simulink model "ssc_auto_ev_20b"  (R2020b)
settings: Solver=VariableStepAuto  StartTime=0.0  StopTime=200  RelTol=1e-3  AbsTol=1e-3
PreLoadFcn:
  | % Simulation parameters
  | dt = 0.01;
  | 
  | % Battery cell parameters
  | ssc_lithium_cell_1RC_ini
  | Nseries = 100;
  | Nparallel = 10;
  | 
  | % Motor parameters
  | max_torque = 220;
  | max_power = 80e3;
  | 
  | % Vehicle parameters
  | vehicle_mass = 4000;
  | wheel_radius = 0.35;
  | area = 5;
  | drag_coefficient = 0.25;
  | air_density = 1.225;
  | gravity = 9.81;
  | rolling_res_ratio = 0.015;
  | 
  | % Differential drive parameters
  | gear_ratio = 12;
  | 
  | % Simplified braking system parameters
  | force_max_pedal = 500;
  | braking_torque_to_pedal_force_ratio = -16;
  | 
  | % Vehicle controller parameters
  | hill_hold_max_speed = 0.5;
  | 
  | % Water properties for cooling circuit
  | load WaterProperties
  | 
  | % Input signals for Signal Editor block
  | load ssc_auto_ev_Inputs
values from neighbouring files (symbols this model uses):
  C1_LUT = [1913.6 4625.7 23306 10736 18036 12251 9022.9 12447 18872 40764 18721 33630 ... (21 elements, 7x3)]    [ssc_auto_ev_param.mat]
  Capacity_LUT = [28.0081 27.625 27.6392]    [ssc_auto_ev_param.mat]
  cell_Cp_heat = 810.5328    [ssc_auto_ev_param.mat]
  cell_mass = 1    [ssc_auto_ev_param.mat]
  Em_LUT = [3.4966 3.5519 3.6183 3.7066 3.9131 4.0748 4.1923 3.5057 3.566 3.6337 3.7127 3.9259 ... (21 elements, 7x3)]    [ssc_auto_ev_param.mat]
  Qe_init = 15.6845    [ssc_auto_ev_param.mat]
  R0_LUT = [0.0117 0.011 0.0114 0.0107 0.0107 0.0113 0.0116 0.0085 0.0085 0.0087 0.0082 0.0083 ... (21 elements, 7x3)]    [ssc_auto_ev_param.mat]
  R1_LUT = [0.0109 0.0069 0.0047 0.0034 0.0033 0.0033 0.0028 0.0029 0.0024 0.0026 0.0016 0.0023 ... (21 elements, 7x3)]    [ssc_auto_ev_param.mat]
  SOC_LUT = [0 0.1 0.25 0.5 0.75 0.9 1]    [ssc_auto_ev_param.mat]
  T_init = 293.15    [ssc_auto_ev_param.mat]
  Temperature_LUT = [278.15 293.15 313.15]    [ssc_auto_ev_param.mat]
undefined symbols (not defined in the file or in its folder): DiscIntNeverNeededParam, K, Lambda, tau, x0
libraries: fl_lib x656, nesl_utility x86, simulink x21, LiBatteryElements_lib x16, SignalEditorBlockLib x4, simulink_extras x4
(part 11 of 13)

== system ssc_auto_ev_20b/Step 3: Ungroup and Redraw/Port 1 Interface1/Interface/Continuous ==
  through2 : Inport
  through1 : Inport  Port=2
  1/thermalMass : Gain  Gain=1/thermalMass  SaturateOnIntegerOverflow=on  OutDataTypeStr=Inherit: Same as input  ParamDataTypeStr=Inherit: Same as input
  Integrator : Integrator  InitialCondition=T0
  Prediction : Subsystem  Commented=through  mask(Prediction (discrete->continuous)){h2=h2}
      mask prompts: h2 "physmod:simscape:couplers:SimscapeNetworkCouplersLib:PortUDiscreteSampleTimes_MP"
      mask help: physmod:simscape:couplers:SimscapeNetworkCouplersLib:Predictiondiscretecontinuous_MD
  Smoothing : Subsystem  Commented=through  mask(Smoothing (continuous->discrete)){tsSmoothing=tsSmoothing, smoothing0=T0}
      mask prompts: tsSmoothing "physmod:simscape:couplers:SimscapeNetworkCouplersLib:SmoothingTimeConstants_MP"; smoothing0 "physmod:simscape:couplers:SimscapeNetworkCouplersLib:InitialOutput_MP"
      mask help: physmod:simscape:couplers:SimscapeNetworkCouplersLib:Smoothingcontinuousdiscrete_MD
  Sum : Sum  InputSameDT=on  SaturateOnIntegerOverflow=on  OutDataTypeStr=Inherit: Same as first input
  across2 : Outport
  across1 : Outport  Port=2
  wires:
  Integrator/1 -> Smoothing/1(u), across1/1
  1/thermalMass/1 -> Integrator/1
  Sum/1 -> 1/thermalMass/1
  Smoothing/1(y) -> across2/1
  Prediction/1(y) -> Sum/2
  through1/1 -> Sum/1
  through2/1 -> Prediction/1(u)

== system ssc_auto_ev_20b/Step 3: Ungroup and Redraw/Port 1 Interface1/Interface/Discrete ==
  through2 : Inport
  through1 : Inport  Port=2
  1/thermalMass : Gain  Gain=1/thermalMass  SaturateOnIntegerOverflow=on  OutDataTypeStr=Inherit: Same as input  ParamDataTypeStr=Inherit: Same as input
  Integrator : DiscreteIntegrator  InitialCondition=T0  SampleTime=h1  ICPrevOutput=DiscIntNeverNeededParam  ICPrevScaledInput=DiscIntNeverNeededParam
  Prediction : Subsystem  Commented=through  mask(Prediction (slow->fast)){h2=h2, h1=h1}
      mask prompts: h2 "physmod:simscape:couplers:SimscapeNetworkCouplersLib:PortUDiscreteSampleTimes_MP"; h1 "physmod:simscape:couplers:SimscapeNetworkCouplersLib:PortYDiscreteSampleTimes_MP"
      mask help: physmod:simscape:couplers:SimscapeNetworkCouplersLib:Predictionslowfast_MD
  Smoothing : Subsystem  Commented=through  mask(Smoothing (fast->slow)){nSmooth=nSmooth, h1=h1, smoothing0=T0}
      mask prompts: nSmooth "physmod:simscape:couplers:SimscapeNetworkCouplersLib:NumberOfSamplesOverWhichToSmooth_MP"; h1 "physmod:simscape:couplers:SimscapeNetworkCouplersLib:PortUDiscreteSampleTimes_MP"; smoothing0 "physmod:simscape:couplers:SimscapeNetworkCouplersLib:InitialOutput_MP"
      mask help: physmod:simscape:couplers:SimscapeNetworkCouplersLib:Smoothingfastslow_MD
  Sum : Sum  InputSameDT=on  SaturateOnIntegerOverflow=on  OutDataTypeStr=Inherit: Same as first input
  across2 : Outport
  across1 : Outport  Port=2
  wires:
  1/thermalMass/1 -> Integrator/1
  Sum/1 -> 1/thermalMass/1
  Integrator/1 -> Smoothing/1(u), across1/1
  Smoothing/1(y) -> across2/1
  Prediction/1(y) -> Sum/2
  through2/1 -> Prediction/1(u)
  through1/1 -> Sum/1

== system ssc_auto_ev_20b/Step 3: Ungroup and Redraw/Port 1 Interface2/Interface/Continuous ==
  through2 : Inport
  through1 : Inport  Port=2
  1/thermalMass : Gain  Gain=1/thermalMass  SaturateOnIntegerOverflow=on  OutDataTypeStr=Inherit: Same as input  ParamDataTypeStr=Inherit: Same as input
  Integrator : Integrator  InitialCondition=T0
  Prediction : Subsystem  Commented=through  mask(Prediction (discrete->continuous)){h2=h2}
      mask prompts: h2 "physmod:simscape:couplers:SimscapeNetworkCouplersLib:PortUDiscreteSampleTimes_MP"
      mask help: physmod:simscape:couplers:SimscapeNetworkCouplersLib:Predictiondiscretecontinuous_MD
  Smoothing : Subsystem  Commented=through  mask(Smoothing (continuous->discrete)){tsSmoothing=tsSmoothing, smoothing0=T0}
      mask prompts: tsSmoothing "physmod:simscape:couplers:SimscapeNetworkCouplersLib:SmoothingTimeConstants_MP"; smoothing0 "physmod:simscape:couplers:SimscapeNetworkCouplersLib:InitialOutput_MP"
      mask help: physmod:simscape:couplers:SimscapeNetworkCouplersLib:Smoothingcontinuousdiscrete_MD
  Sum : Sum  InputSameDT=on  SaturateOnIntegerOverflow=on  OutDataTypeStr=Inherit: Same as first input
  across2 : Outport
  across1 : Outport  Port=2
  wires:
  through2/1 -> Prediction/1(u)
  through1/1 -> Sum/1
  Prediction/1(y) -> Sum/2
  Smoothing/1(y) -> across2/1
  Sum/1 -> 1/thermalMass/1
  1/thermalMass/1 -> Integrator/1
  Integrator/1 -> across1/1, Smoothing/1(u)

== system ssc_auto_ev_20b/Step 3: Ungroup and Redraw/Port 1 Interface2/Interface/Discrete ==
  through2 : Inport
  through1 : Inport  Port=2
  1/thermalMass : Gain  Gain=1/thermalMass  SaturateOnIntegerOverflow=on  OutDataTypeStr=Inherit: Same as input  ParamDataTypeStr=Inherit: Same as input
  Integrator : DiscreteIntegrator  InitialCondition=T0  SampleTime=h1  ICPrevOutput=DiscIntNeverNeededParam  ICPrevScaledInput=DiscIntNeverNeededParam
  Prediction : Subsystem  Commented=through  mask(Prediction (slow->fast)){h2=h2, h1=h1}
      mask prompts: h2 "physmod:simscape:couplers:SimscapeNetworkCouplersLib:PortUDiscreteSampleTimes_MP"; h1 "physmod:simscape:couplers:SimscapeNetworkCouplersLib:PortYDiscreteSampleTimes_MP"
      mask help: physmod:simscape:couplers:SimscapeNetworkCouplersLib:Predictionslowfast_MD
  Smoothing : Subsystem  Commented=through  mask(Smoothing (fast->slow)){nSmooth=nSmooth, h1=h1, smoothing0=T0}
      mask prompts: nSmooth "physmod:simscape:couplers:SimscapeNetworkCouplersLib:NumberOfSamplesOverWhichToSmooth_MP"; h1 "physmod:simscape:couplers:SimscapeNetworkCouplersLib:PortUDiscreteSampleTimes_MP"; smoothing0 "physmod:simscape:couplers:SimscapeNetworkCouplersLib:InitialOutput_MP"
      mask help: physmod:simscape:couplers:SimscapeNetworkCouplersLib:Smoothingfastslow_MD
  Sum : Sum  InputSameDT=on  SaturateOnIntegerOverflow=on  OutDataTypeStr=Inherit: Same as first input
  across2 : Outport
  across1 : Outport  Port=2
  wires:
  through1/1 -> Sum/1
  through2/1 -> Prediction/1(u)
  Prediction/1(y) -> Sum/2
  Smoothing/1(y) -> across2/1
  Integrator/1 -> across1/1, Smoothing/1(u)
  Sum/1 -> 1/thermalMass/1
  1/thermalMass/1 -> Integrator/1

== system ssc_auto_ev_20b/Step 3: Ungroup and Redraw/Port 1 Interface3/Interface/Continuous ==
  across2 : Inport
  through1 : Inport  Port=2
  -1 : Gain  Gain=-1  SaturateOnIntegerOverflow=on  OutDataTypeStr=Inherit: Same as input  ParamDataTypeStr=Inherit: Same as input
  1/tau : Gain  Gain=1/tau  SaturateOnIntegerOverflow=on  OutDataTypeStr=Inherit: Same as input  ParamDataTypeStr=Inherit: Same as input
  1/tau1 : Gain  Gain=1/tau  SaturateOnIntegerOverflow=on  OutDataTypeStr=Inherit: Same as input  ParamDataTypeStr=Inherit: Same as input
  Integrator : Integrator  InitialCondition=i0
  Integrator1 : Integrator  InitialCondition=v0
  Prediction : Subsystem  Commented=through  mask(Prediction (discrete->continuous)){h2=h2}
      mask prompts: h2 "physmod:simscape:couplers:SimscapeNetworkCouplersLib:PortUDiscreteSampleTimes_MP"
      mask help: physmod:simscape:couplers:SimscapeNetworkCouplersLib:Predictiondiscretecontinuous_MD
  Smoothing : Subsystem  Commented=through  mask(Smoothing (continuous->discrete)){tsSmoothing=tsSmoothing, smoothing0=i0}
      mask prompts: tsSmoothing "physmod:simscape:couplers:SimscapeNetworkCouplersLib:SmoothingTimeConstants_MP"; smoothing0 "physmod:simscape:couplers:SimscapeNetworkCouplersLib:InitialOutput_MP"
      mask help: physmod:simscape:couplers:SimscapeNetworkCouplersLib:Smoothingcontinuousdiscrete_MD
  Sum : Sum  Inputs=|+-  InputSameDT=on  SaturateOnIntegerOverflow=on  OutDataTypeStr=Inherit: Same as first input
  Sum1 : Sum  Inputs=|+-  InputSameDT=on  SaturateOnIntegerOverflow=on  OutDataTypeStr=Inherit: Same as first input
  through2 : Outport
  across1 : Outport  Port=2
  wires:
  across2/1 -> Prediction/1(u)
  Smoothing/1(y) -> -1/1
  1/tau/1 -> Integrator/1
  Sum/1 -> 1/tau/1
  Integrator/1 -> Smoothing/1(u), Sum/2
  through1/1 -> Sum/1
  Integrator1/1 -> Sum1/2, across1/1
  1/tau1/1 -> Integrator1/1
  Sum1/1 -> 1/tau1/1
  Prediction/1(y) -> Sum1/1
  -1/1 -> through2/1

== system ssc_auto_ev_20b/Step 3: Ungroup and Redraw/Port 1 Interface3/Interface/Discrete ==
  across2 : Inport
  through1 : Inport  Port=2
  -1 : Gain  Gain=-1  SaturateOnIntegerOverflow=on  OutDataTypeStr=Inherit: Same as input  ParamDataTypeStr=Inherit: Same as input
  1/tau : Gain  Gain=1/tau  SaturateOnIntegerOverflow=on  OutDataTypeStr=Inherit: Same as input  ParamDataTypeStr=Inherit: Same as input
  1/tau1 : Gain  Gain=1/tau  SaturateOnIntegerOverflow=on  OutDataTypeStr=Inherit: Same as input  ParamDataTypeStr=Inherit: Same as input
  Integrator/1 : DiscreteIntegrator  InitialCondition=v0  SampleTime=h1  ICPrevOutput=DiscIntNeverNeededParam  ICPrevScaledInput=DiscIntNeverNeededParam
  Integrator/2 : DiscreteIntegrator  InitialCondition=i0  SampleTime=h1  ICPrevOutput=DiscIntNeverNeededParam  ICPrevScaledInput=DiscIntNeverNeededParam
  Prediction : Subsystem  Commented=through  mask(Prediction (slow->fast)){h2=h2, h1=h1}
      mask prompts: h2 "physmod:simscape:couplers:SimscapeNetworkCouplersLib:PortUDiscreteSampleTimes_MP"; h1 "physmod:simscape:couplers:SimscapeNetworkCouplersLib:PortYDiscreteSampleTimes_MP"
      mask help: physmod:simscape:couplers:SimscapeNetworkCouplersLib:Predictionslowfast_MD
  Smoothing : Subsystem  Commented=through  mask(Smoothing (fast->slow)){nSmooth=nSmooth, h1=h1, smoothing0=i0}
      mask prompts: nSmooth "physmod:simscape:couplers:SimscapeNetworkCouplersLib:NumberOfSamplesOverWhichToSmooth_MP"; h1 "physmod:simscape:couplers:SimscapeNetworkCouplersLib:PortUDiscreteSampleTimes_MP"; smoothing0 "physmod:simscape:couplers:SimscapeNetworkCouplersLib:InitialOutput_MP"
      mask help: physmod:simscape:couplers:SimscapeNetworkCouplersLib:Smoothingfastslow_MD
  Sum : Sum  Inputs=|+-  InputSameDT=on  SaturateOnIntegerOverflow=on  OutDataTypeStr=Inherit: Same as first input
  Sum1 : Sum  Inputs=|+-  InputSameDT=on  SaturateOnIntegerOverflow=on  OutDataTypeStr=Inherit: Same as first input
  through2 : Outport
  across1 : Outport  Port=2
  wires:
  across2/1 -> Prediction/1(u)
  Smoothing/1(y) -> -1/1
  Prediction/1(y) -> Sum1/1
  Sum1/1 -> 1/tau1/1
  Integrator/1/1 -> across1/1, Sum1/2
  Integrator/2/1 -> Smoothing/1(u), Sum/2
  Sum/1 -> 1/tau/1
  1/tau1/1 -> Integrator/1/1
  1/tau/1 -> Integrator/2/1
  through1/1 -> Sum/1
  -1/1 -> through2/1

== system ssc_auto_ev_20b/Step 3: Ungroup and Redraw/Vehicle Dynamics/Brake Torque/Smooth Sign ==
  1 : fl_lib/Physical Signals/Sources/PS Constant  constant=1
      settings: SourceProductBaseCode=PW,SS,VE
  2 : fl_lib/Physical Signals/Functions/PS Gain  gain=2 1/(rad/s)
      settings: SourceProductBaseCode=PW,SS,VE
  PS Add : fl_lib/Physical Signals/Functions/PS Add
      settings: SourceProductBaseCode=PW,SS,VE
  PS Subtract : fl_lib/Physical Signals/Functions/PS Subtract
      settings: SourceProductBaseCode=PW,SS,VE
  exp(2x) : fl_lib/Physical Signals/Functions/PS Math Function  fcn_choice=foundation.enum.math_function.exp
      settings: SourceProductBaseCode=PW,SS,VE
  tanh(x) : fl_lib/Physical Signals/Functions/PS Divide
      settings: SourceProductBaseCode=PW,SS,VE
  x : PMIOPort  Side=Left
  y : PMIOPort  Port=2  Side=Right
  connections:
  tanh(x)/RConn1 -- y/RConn1
  2/LConn1 -- x/RConn1
  tanh(x)/LConn1 -- PS Subtract/RConn1
  tanh(x)/LConn2 -- PS Add/RConn1
  PS Add/LConn2 -- PS Subtract/LConn1 -- exp(2x)/RConn1
  exp(2x)/LConn1 -- 2/RConn1
  PS Add/LConn1 -- PS Subtract/LConn2 -- 1/RConn1

== system ssc_auto_ev_20b/Step 3: Ungroup and Redraw/Vehicle Control/Cruise Control/Capture speed ==
  In1 : Inport
  Trigger : TriggerPort  VariantControl=Variant
  Out1 : Outport  VectorParamsAs1DForOutWhenUnconnected=off
  wires:
  In1/1 -> Out1/1

== system ssc_auto_ev_20b/Step 3: Ungroup and Redraw/Vehicle Control/Cruise Control/Speed Controller ==
  wRef : Inport
  wMeas : Inport  Port=2
  Add : Sum  Inputs=|+-
  Add1 : Sum
  Discrete-Time Integrator : DiscreteIntegrator  gainval=Ki  SampleTime=ts  LimitOutput=on  UpperSaturationLimit=trqMax  LowerSaturationLimit=-trqMax  ICPrevOutput=DiscIntNeverNeededParam  ICPrevScaledInput=DiscIntNeverNeededParam
  Kp : Gain  Gain=Kp
  trqRef : Outport  VectorParamsAs1DForOutWhenUnconnected=off
  wires:
  wRef/1 -> Add/1
  Kp/1 -> Add1/1
  Discrete-Time Integrator/1 -> Add1/2
  wMeas/1 -> Add/2
  Add1/1 -> trqRef/1
  Add/1 -> Kp/1, Discrete-Time Integrator/1

== system ssc_auto_ev_20b/Step 4: Deployment Model/Battery @50Hz/Battery/Electric and Thermal Model ==
  note: Equivalent Circuit Model for Single Battery Cell
  C1 : LiBatteryElements_lib/C_table  C_Table=C1_LUT*Nparallel F  SOC_Table=SOC_LUT  Temp_Table=Temperature_LUT K  v0=0 V
      settings: SourceProductBaseCode=SS  InternalSimscapePortConfiguration="{\"Bottom\":[],\"Left\":[{\"id\":\"p\",\"label\":\"+\",\"type\":\"foundation.electrical.electrical\"},{\"id\":\"T\",\"label\":\"T\",\"type\":\"input\"},{\"id\":\"SOC\",\"label\":\"SOC\",\"type\":\"input\"}],\"Right\":[{\"id\":\"n\",\"label\":\"-\",\"type\":\"foundation.electrical.electrical\"}],\"Top\":[]}"
  Em_table : LiBatteryElements_lib/Em_table  C_Table=Capacity_LUT*Nparallel hr*A  Em_Table=Em_LUT V  SOC_Table=SOC_LUT  Temp_Table=Temperature_LUT K  Qinit=Qe_init*Nparallel hr*A
      settings: SourceProductBaseCode=SS  InternalSimscapePortConfiguration="{\"Bottom\":[],\"Left\":[{\"id\":\"p\",\"label\":\"+\",\"type\":\"foundation.electrical.electrical\"},{\"id\":\"C\",\"label\":\"C\",\"type\":\"output\"},{\"id\":\"SOC\",\"label\":\"SOC\",\"type\":\"output\"}],\"Right\":[{\"id\":\"n\",\"label\":\"-\",\"type\":\"foundation.electrical.electrical\"},{\"id\":\"T\",\"label\":\"T\",\"type\":\"input\"}],\"Top\":[]}"
  NumCells : fl_lib/Physical Signals/Functions/PS Gain  gain=Nseries
      settings: SourceProductBaseCode=PW,SS,VE
  PS Add : fl_lib/Physical Signals/Functions/PS Add
      settings: SourceProductBaseCode=PW,SS,VE
  R0 : LiBatteryElements_lib/R_table  R_Table=R0_LUT/Nparallel Ohm  SOC_Table=SOC_LUT  Temp_Table=Temperature_LUT K
      settings: SourceProductBaseCode=SS  InternalSimscapePortConfiguration="{\"Bottom\":[],\"Left\":[{\"id\":\"p\",\"label\":\"+\",\"type\":\"foundation.electrical.electrical\"},{\"id\":\"T\",\"label\":\"T\",\"type\":\"input\"},{\"id\":\"SOC\",\"label\":\"SOC\",\"type\":\"input\"}],\"Right\":[{\"id\":\"n\",\"label\":\"-\",\"type\":\"foundation.electrical.electrical\"},{\"id\":\"pow\",\"label\":\"POW\",\"type\":\"output\"}],\"Top\":[]}"
  R1 : LiBatteryElements_lib/R_table  R_Table=R1_LUT/Nparallel Ohm  SOC_Table=SOC_LUT  Temp_Table=Temperature_LUT K
      settings: SourceProductBaseCode=SS  InternalSimscapePortConfiguration="{\"Bottom\":[],\"Left\":[{\"id\":\"p\",\"label\":\"+\",\"type\":\"foundation.electrical.electrical\"},{\"id\":\"T\",\"label\":\"T\",\"type\":\"input\"},{\"id\":\"SOC\",\"label\":\"SOC\",\"type\":\"input\"}],\"Right\":[{\"id\":\"n\",\"label\":\"-\",\"type\":\"foundation.electrical.electrical\"},{\"id\":\"pow\",\"label\":\"POW\",\"type\":\"output\"}],\"Top\":[]}"
  Thermal Model : Subsystem
  + : PMIOPort  Side=Right
  - : PMIOPort  Port=2  Side=Right
  H : PMIOPort  Tag=PMCPort  Port=3  Side=Left
  connections:
  PS Add/RConn1 -- NumCells/LConn1
  +/RConn1 -- R0/RConn1
  C1/LConn2 -- R0/LConn2 -- Em_table/RConn2 -- Thermal Model/RConn1 -- R1/LConn2
  Em_table/LConn1 -- R1/LConn1 -- C1/LConn1
  PS Add/LConn2 -- R1/RConn2
  PS Add/LConn1 -- R0/RConn2
  C1/RConn1 -- R1/RConn1 -- R0/LConn1
  Em_table/RConn1 -- -/RConn1
  R0/LConn3 -- Em_table/LConn3 -- C1/LConn3 -- R1/LConn3
  NumCells/RConn1 -- Thermal Model/LConn1
  H/RConn1 -- Thermal Model/LConn2

== system ssc_auto_ev_20b/Step 4: Deployment Model/Battery @50Hz/Port 1 Interface/Interface ==
  through1 : Inport
  through2 : Inport  Port=2
  Continuous : Subsystem  VariantControl=Continuous
  Discrete : Subsystem  VariantControl=Discrete
  across2 : Outport
  across1 : Outport  Port=2

== system ssc_auto_ev_20b/Step 4: Deployment Model/Control @100Hz/Driver and Environment/Bus ==
  In : Inport
  Wi : Inport  Port=2
  Br : Inport  Port=3
  Bus Creator : BusCreator  Inputs=3
  b : Outport  VectorParamsAs1DForOutWhenUnconnected=off
  wires:
  Wi/1 -> Bus Creator/2  "Wind speed"
  Bus Creator/1 -> b/1
  Br/1 -> Bus Creator/3  "Brake pedal"
  In/1 -> Bus Creator/1  "Incline"

== system ssc_auto_ev_20b/Step 4: Deployment Model/Control @100Hz/Driver and Environment/Inclinometer ==
  a : Inport
  Trigonometric Function : Trigonometry
  d2r : Gain  Gain=pi/180
  g : Gain  Gain=gravity
  y : Outport  VectorParamsAs1DForOutWhenUnconnected=off
  wires:
  Trigonometric Function/1 -> g/1
  a/1 -> d2r/1
  d2r/1 -> Trigonometric Function/1
  g/1 -> y/1

== system ssc_auto_ev_20b/Step 4: Deployment Model/Control @100Hz/Vehicle Control/Cruise Control ==
  Enable : Inport
  Disable : Inport  Port=2
  wMeas : Inport  Port=3
  Brake sw : Inport  Port=4
  Capture speed : Subsystem  TreatAsAtomicUnit=on
  Data Type Conversion1 : DataTypeConversion  OutDataTypeStr=boolean
  J-K Flip-Flop : simulink_extras/Flip Flops/J-K Flip-Flop  initial_condition=0
  Logical Operator : Logic  Operator=OR  AllPortsSameDT=off  OutDataTypeStr=boolean
  Pulse Generator : DiscretePulseGenerator  Period=10  PulseWidth=5  SampleTime=0.01
  Speed Controller : Subsystem  mask(P+I motor speed controller){Kp=100, Ki=100, trqMax=max_torque, ts=dt}
      mask prompts: Kp "Proportional gain (Nm/(rad/s))"; Ki "Integral gain (Nm/rad)"; trqMax "Maximum torque demand"; ts "Sample time"
      mask help: Inputs wRef and wMeas are the demanded rotor speed and measured rotor speed in rad/s. The controller output is a torque demand in Nm.
  Terminator : Terminator
  trqRef : Outport  VectorParamsAs1DForOutWhenUnconnected=off
  Enabled : Outport  Port=2  VectorParamsAs1DForOutWhenUnconnected=off
  wires:
  Enable/1 -> Data Type Conversion1/1
  Pulse Generator/1 -> J-K Flip-Flop/2
  Disable/1 -> Logical Operator/1
  Speed Controller/1(trqRef) -> trqRef/1
  Brake sw/1 -> Logical Operator/2
  wMeas/1 -> Capture speed/1(In1), Speed Controller/2(wMeas)
  Logical Operator/1 -> J-K Flip-Flop/3
  J-K Flip-Flop/1 -> Enabled/1, Capture speed/Trigger
  Data Type Conversion1/1 -> J-K Flip-Flop/1
  J-K Flip-Flop/2 -> Terminator/1
  Capture speed/1(Out1) -> Speed Controller/1(wRef)

== system ssc_auto_ev_20b/Step 4: Deployment Model/Control @100Hz/Vehicle Control/Feedforward term for regenerative braking on downhill ==
  Inclin. : Inport
  " M " : Gain  Gain=vehicle_mass
  1/ratio : Gain  Gain=1/gear_ratio
  Two motors : Gain  Gain=0.5
  Wheel radius : Gain  Gain=wheel_radius
  "[-inf,0]" : Saturate  UpperLimit=0  LowerLimit=-inf
  Feedfwd trq : Outport  VectorParamsAs1DForOutWhenUnconnected=off
  wires:
  Two motors/1 -> Feedfwd trq/1
  1/ratio/1 -> Two motors/1  "Motor torque"
  "[-inf,0]"/1 -> " M "/1
  Inclin./1 -> "[-inf,0]"/1
  " M "/1 -> Wheel radius/1
  Wheel radius/1 -> 1/ratio/1  "Wheel torque"

== system ssc_auto_ev_20b/Step 4: Deployment Model/Control @100Hz/Vehicle Control/Max Power ==
  Vspd : Inport
  Abs : Abs
  Constant : Constant
  Math Function : Math  Operator=reciprocal  SignedPower=on  SaturateOnIntegerOverflow=on
  Prevent divide by zero : Switch  Criteria=u2 > Threshold  Threshold=1
  max_power : Gain  Gain=max_power
  Max Power : Outport  VectorParamsAs1DForOutWhenUnconnected=off
  wires:
  Prevent divide by zero/1 -> Math Function/1
  Constant/1 -> Prevent divide by zero/3
  Abs/1 -> Prevent divide by zero/2, Prevent divide by zero/1
  Math Function/1 -> max_power/1
  max_power/1 -> Max Power/1
  Vspd/1 -> Abs/1

== system ssc_auto_ev_20b/Step 4: Deployment Model/Control @100Hz/Vehicle Control/Torque Demand Management ==
  Brake : Inport
  Throttle : Inport  Port=2
  wMeas : Inport  Port=3
  FFbrake : Inport  Port=4
  1/ratio : Gain  Gain=1/gear_ratio
  Disable braking at low and negative speeds : Lookup_n-D  NumberOfTableDimensions=1  BreakpointsForDimension1=[-100 -1 0 5 10 100]  Table=[0 0 0 0 1 1]  InternalRulePriority=Speed  RndMeth=Simplest  InputSameDT=on
  Disable braking at low and negative speeds1 : Lookup_n-D  NumberOfTableDimensions=1  BreakpointsForDimension1=[-100 -1 0 5 10 100]  Table=[0 0 0 0 1 1]  InternalRulePriority=Speed  RndMeth=Simplest  InputSameDT=on
  Force for max pedal deflection : Gain  Gain=force_max_pedal
  Max torque demand : Gain  Gain=max_torque
  Motor torque limits2 : Saturate  UpperLimit=max_torque  LowerLimit=-max_torque
  Product : Product
  Product1 : Product
  Sum : Sum  Inputs=|++
  Sum1 : Sum  Inputs=|++
  Torque per unit brake pedal force : Gain  Gain=braking_torque_to_pedal_force_ratio
  Two motors : Gain  Gain=1/2
  wMeas1 : InportShadow  Port=3
  Dem trq : Outport  VectorParamsAs1DForOutWhenUnconnected=off
  wires:
  Motor torque limits2/1 -> Dem trq/1
  Sum1/1 -> Motor torque limits2/1
  Product1/1 -> Sum1/2
  wMeas1/1 -> Disable braking at low and negative speeds1/1
  Disable braking at low and negative speeds1/1 -> Product1/2
  FFbrake/1 -> Product1/1
  Disable braking at low and negative speeds/1 -> Product/2
  Sum/1 -> Sum1/1
  Max torque demand/1 -> Sum/1
  Brake/1 -> Force for max pedal deflection/1
  Throttle/1 -> Max torque demand/1
  Torque per unit brake pedal force/1 -> 1/ratio/1
  1/ratio/1 -> Two motors/1
  Force for max pedal deflection/1 -> Torque per unit brake pedal force/1
  wMeas/1 -> Disable braking at low and negative speeds/1
  Product/1 -> Sum/2
  Two motors/1 -> Product/1

== system ssc_auto_ev_20b/Step 4: Deployment Model/Thermal @20Hz/Cooling System/ Heat Exchanger Characteristic ==
  Characteristic : Subsystem
  Heat Flow Source : fl_lib/Thermal/Thermal Sources/Controlled Heat Flow Rate Source
      settings: SourceProductBaseCode=PW,SS,VE
  Mass Flow Rate & Thermal Flux Sensor (TL) : fl_lib/Thermal Liquid/Sensors/Mass & Energy Flow Rate Sensor (TL)
      settings: SourceProductBaseCode=PW,SS,VE  InternalSimscapePortConfiguration="{\"Bottom\":[],\"Left\":[{\"id\":\"A\",\"label\":\"A\",\"type\":\"foundation.thermal_liquid.thermal_liquid\"}],\"Right\":[{\"id\":\"B\",\"label\":\"B\",\"type\":\"foundation.thermal_liquid.thermal_liquid\"},{\"id\":\"M\",\"label\":\"M\",\"type\":\"output\"},{\"id\":\"PHI\",\"label\":\"Phi\",\"type\":\"output\"}],\"Top\":[]}"
  Temperature Sensor : fl_lib/Thermal/Thermal Sensors/Temperature Sensor
      settings: SourceProductBaseCode=PW,SS,VE
  ThRef : fl_lib/Thermal/Thermal Elements/Thermal Reference
      settings: SourceProductBaseCode=PW,SS,VE
  Henv : PMIOPort  Side=Right
  Hp : PMIOPort  Port=2  Side=Left
  B : PMIOPort  Port=3  Side=Right
  Phi : PMIOPort  Port=4  Side=Right
  A : PMIOPort  Port=5  Side=Left
  T in : PMIOPort  Port=6  Side=Left
  connections:
  A/RConn1 -- Mass Flow Rate & Thermal Flux Sensor (TL)/LConn1
  Temperature Sensor/LConn1 -- Henv/RConn1 -- Heat Flow Source/RConn2
  ThRef/LConn1 -- Temperature Sensor/RConn1
  Heat Flow Source/LConn1 -- Hp/RConn1
  Mass Flow Rate & Thermal Flux Sensor (TL)/RConn1 -- B/RConn1
  Mass Flow Rate & Thermal Flux Sensor (TL)/RConn3 -- Phi/RConn1
  Mass Flow Rate & Thermal Flux Sensor (TL)/RConn2 -- Characteristic/RConn1
  T in/RConn1 -- Characteristic/RConn2
  Temperature Sensor/RConn2 -- Characteristic/RConn3
  Characteristic/LConn1 -- Heat Flow Source/RConn1

== system ssc_auto_ev_20b/Step 4: Deployment Model/Thermal @20Hz/Cooling System/Expansion Tank ==
  Air Stiffness : fl_lib/Mechanical/Translational Elements/Translational Spring  spr_rate=1e3 N/m  v_specify=off  v_priority=High  v=0 m/s  v_nominal_specify=off  v_nominal_unit=m/s  v_nominal_value=1  f_specify=on  f_priority=Low  f=0 N  f_nominal_specify=off  f_nominal_unit=N  f_nominal_value=1  x_specify=off  x_priority=High  x=0 m  x_nominal_specify=off  x_nominal_unit=m  x_nominal_value=1
      settings: SourceProductBaseCode=PW,SS,VE
  Expansion Tank : fl_lib/Thermal Liquid/Elements/Translational Mechanical Converter (TL)  mech_orientation=1  interface_area=pi*50^2 mm^2  x0=200 mm  dead_volume=0.001 m^3  environment_spec=1  environment_pressure=0.101325 MPa  dynamic_compressibility=0  p0=1 atm  T0=20 degC
      settings: SourceProductBaseCode=PW,SS,VE  InternalSimscapePortConfiguration="{\"Bottom\":[],\"Left\":[{\"id\":\"A\",\"label\":\"A\",\"type\":\"foundation.thermal_liquid.thermal_liquid\"},{\"id\":\"C\",\"label\":\"C\",\"type\":\"foundation.mechanical.translational.translational\"},{\"id\":\"H\",\"label\":\"H\",\"type\":\"foundation.thermal.thermal\"}],\"Right\":[{\"id\":\"R\",\"label\":\"R\",\"type\":\"foundation.mechanical.translational.translational\"}],\"Top\":[]}"
  Expansion Tank Inlet : fl_lib/Thermal Liquid/Elements/Local Restriction (TL)  restriction_type=foundation.enum.restriction_type.fixed  restriction_area=pi*10^2 mm^2  min_area=1e-10 m^2  max_area=0.005 m^2  area=pi*11^2 mm^2  Cd=0.7  pressure_recovery=0  Re_c=12
      settings: SourceProductBaseCode=PW,SS,VE
  Insulator Expansion Tank : fl_lib/Thermal/Thermal Elements/Perfect Insulator  T_specify=off  T_priority=High  T=0 K  T_nominal_specify=off  T_nominal_unit=K  T_nominal_value=1
      settings: SourceProductBaseCode=PW,SS,VE
  MTRef : fl_lib/Mechanical/Translational Elements/Mechanical Translational Reference
      settings: SourceProductBaseCode=PW,SS,VE
  MTRef Air Stiffness : fl_lib/Mechanical/Translational Elements/Mechanical Translational Reference
      settings: SourceProductBaseCode=PW,SS,VE
  A : PMIOPort  Side=Left
  connections:
  Air Stiffness/RConn1 -- MTRef Air Stiffness/LConn1
  Air Stiffness/LConn1 -- Expansion Tank/RConn1
  Expansion Tank Inlet/RConn1 -- Expansion Tank/LConn1
  Expansion Tank Inlet/LConn1 -- A/RConn1
  Insulator Expansion Tank/LConn1 -- Expansion Tank/LConn3
  MTRef/LConn1 -- Expansion Tank/LConn2

== system ssc_auto_ev_20b/Step 4: Deployment Model/Thermal @20Hz/Cooling System/Heat Exchanger Characteristic ==
  Characteristic : Subsystem
  Heat Flow Source : fl_lib/Thermal/Thermal Sources/Controlled Heat Flow Rate Source
      settings: SourceProductBaseCode=PW,SS,VE
  Mass Flow Rate & Thermal Flux Sensor (TL) : fl_lib/Thermal Liquid/Sensors/Mass & Energy Flow Rate Sensor (TL)
      settings: SourceProductBaseCode=PW,SS,VE  InternalSimscapePortConfiguration="{\"Bottom\":[],\"Left\":[{\"id\":\"A\",\"label\":\"A\",\"type\":\"foundation.thermal_liquid.thermal_liquid\"}],\"Right\":[{\"id\":\"B\",\"label\":\"B\",\"type\":\"foundation.thermal_liquid.thermal_liquid\"},{\"id\":\"M\",\"label\":\"M\",\"type\":\"output\"},{\"id\":\"PHI\",\"label\":\"Phi\",\"type\":\"output\"}],\"Top\":[]}"
  Temperature Sensor : fl_lib/Thermal/Thermal Sensors/Temperature Sensor
      settings: SourceProductBaseCode=PW,SS,VE
  ThRef : fl_lib/Thermal/Thermal Elements/Thermal Reference
      settings: SourceProductBaseCode=PW,SS,VE
  HMotor : PMIOPort  Side=Right
  B : PMIOPort  Port=2  Side=Right
  Hp : PMIOPort  Port=3  Side=Left
  A : PMIOPort  Port=4  Side=Left
  TIn : PMIOPort  Port=5  Side=Left
  connections:
  Mass Flow Rate & Thermal Flux Sensor (TL)/RConn1 -- B/RConn1
  Heat Flow Source/RConn2 -- Temperature Sensor/LConn1 -- HMotor/RConn1
  ThRef/LConn1 -- Temperature Sensor/RConn1
  Heat Flow Source/LConn1 -- Hp/RConn1
  A/RConn1 -- Mass Flow Rate & Thermal Flux Sensor (TL)/LConn1
  Temperature Sensor/RConn2 -- Characteristic/LConn3
  Mass Flow Rate & Thermal Flux Sensor (TL)/RConn2 -- Characteristic/LConn1
  Characteristic/LConn2 -- TIn/RConn1
  Characteristic/RConn1 -- Heat Flow Source/RConn1

== system ssc_auto_ev_20b/Step 4: Deployment Model/Thermal @20Hz/Cooling System/Sensing Inlet Temperature ==
  Pressure & Temperature Sensor (TL) : fl_lib/Thermal Liquid/Sensors/Pressure & Temperature Sensor (TL)
      settings: SourceProductBaseCode=PW,SS,VE  InternalSimscapePortConfiguration="{\"Bottom\":[],\"Left\":[{\"id\":\"A\",\"label\":\"A\",\"type\":\"foundation.thermal_liquid.thermal_liquid\"}],\"Right\":[{\"id\":\"B\",\"label\":\"B\",\"type\":\"foundation.thermal_liquid.thermal_liquid\"},{\"id\":\"P\",\"label\":\"P\",\"type\":\"output\"},{\"id\":\"T\",\"label\":\"T\",\"type\":\"output\"}],\"Top\":[]}"
  TLRef : fl_lib/Thermal Liquid/Elements/Absolute Reference (TL)
      settings: SourceProductBaseCode=PW,SS,VE
  A : PMIOPort  Side=Left
  T : PMIOPort  Port=2  Side=Right
  connections:
  Pressure & Temperature Sensor (TL)/RConn3 -- T/RConn1
  Pressure & Temperature Sensor (TL)/LConn1 -- A/RConn1
  TLRef/LConn1 -- Pressure & Temperature Sensor (TL)/RConn1

== system ssc_auto_ev_20b/Step 4: Deployment Model/Thermal @20Hz/Cooling System/Sensing Temperature ==
  Pressure & Temperature Sensor (TL) : fl_lib/Thermal Liquid/Sensors/Pressure & Temperature Sensor (TL)
      settings: SourceProductBaseCode=PW,SS,VE  InternalSimscapePortConfiguration="{\"Bottom\":[],\"Left\":[{\"id\":\"A\",\"label\":\"A\",\"type\":\"foundation.thermal_liquid.thermal_liquid\"}],\"Right\":[{\"id\":\"B\",\"label\":\"B\",\"type\":\"foundation.thermal_liquid.thermal_liquid\"},{\"id\":\"P\",\"label\":\"P\",\"type\":\"output\"},{\"id\":\"T\",\"label\":\"T\",\"type\":\"output\"}],\"Top\":[]}"
  TLRef : fl_lib/Thermal Liquid/Elements/Absolute Reference (TL)
      settings: SourceProductBaseCode=PW,SS,VE
  T : PMIOPort  Side=Right
  A : PMIOPort  Port=2  Side=Left
  connections:
  Pressure & Temperature Sensor (TL)/RConn3 -- T/RConn1
  TLRef/LConn1 -- Pressure & Temperature Sensor (TL)/RConn1
  A/RConn1 -- Pressure & Temperature Sensor (TL)/LConn1

== system ssc_auto_ev_20b/Step 4: Deployment Model/Vehicle and drive @100Hz/Motor Drive/DC Motor1 ==
  Inertia : fl_lib/Mechanical/Rotational Elements/Inertia  inertia=0.01 kg*m^2  num_ports=foundation.enum.numPorts2.one  w_specify=off  w_priority=High  w=0 rad/s  w_nominal_specify=off  w_nominal_unit=rad/s  w_nominal_value=1  t_specify=off  t_priority=High  t=0 N*m  t_nominal_specify=off  t_nominal_unit=N*m  t_nominal_value=1
      settings: SourceProductBaseCode=PW,SS,VE
  Rotational Electromechanical Converter : fl_lib/Electrical/Electrical Elements/Rotational Electromechanical Converter  K=1 N*m/A  i_specify=off  i_priority=High  i=0 A  i_nominal_specify=off  i_nominal_unit=A  i_nominal_value=1  v_specify=off  v_priority=High  v=0 V  v_nominal_specify=off  v_nominal_unit=V  v_nominal_value=1  t_specify=off  t_priority=High  t=0 N*m  t_nominal_specify=off  t_nominal_unit=N*m  t_nominal_value=1  w_specify=off  w_priority=High  w=0 rad/s  w_nominal_specify=off  w_nominal_unit=rad/s  w_nominal_value=1
      settings: SourceProductBaseCode=PW,SS,VE
  Thermal Resistor : fl_lib/Electrical/Electrical Elements/Thermal Resistor  R0=1 Ohm  T0=298.15 K  alpha=50e-6 1/K  tc=30 s  K_d=100 W/K  T_specify=off  T_priority=High  T=300 K  T_nominal_specify=off  T_nominal_unit=K  T_nominal_value=1
      settings: SourceProductBaseCode=PW,SS,VE  InternalSimscapePortConfiguration="{\"Bottom\":[],\"Left\":[{\"id\":\"H\",\"label\":\"H\",\"type\":\"foundation.thermal.thermal\"},{\"id\":\"p\",\"label\":\"+\",\"type\":\"foundation.electrical.electrical\"}],\"Right\":[{\"id\":\"n\",\"label\":\"-\",\"type\":\"foundation.electrical.electrical\"}],\"Top\":[]}"
  V+ : PMIOPort  Side=Left
  R : PMIOPort  Port=2  Side=Right
  C : PMIOPort  Port=3  Side=Right
  V- : PMIOPort  Port=4  Side=Left
  H : PMIOPort  Port=5  Side=Left
  connections:
  H/RConn1 -- Thermal Resistor/LConn1
  Rotational Electromechanical Converter/RConn2 -- C/RConn1
  R/RConn1 -- Inertia/LConn1 -- Rotational Electromechanical Converter/LConn2
  Rotational Electromechanical Converter/LConn1 -- Thermal Resistor/RConn1
  Thermal Resistor/LConn2 -- V+/RConn1
  V-/RConn1 -- Rotational Electromechanical Converter/RConn1

== system ssc_auto_ev_20b/Step 4: Deployment Model/Vehicle and drive @100Hz/Motor Drive/DC Motor2 ==
  Inertia : fl_lib/Mechanical/Rotational Elements/Inertia  inertia=0.01 kg*m^2  num_ports=foundation.enum.numPorts2.one  w_specify=off  w_priority=High  w=0 rad/s  w_nominal_specify=off  w_nominal_unit=rad/s  w_nominal_value=1  t_specify=off  t_priority=High  t=0 N*m  t_nominal_specify=off  t_nominal_unit=N*m  t_nominal_value=1
      settings: SourceProductBaseCode=PW,SS,VE
  Rotational Electromechanical Converter : fl_lib/Electrical/Electrical Elements/Rotational Electromechanical Converter  K=1 N*m/A  i_specify=off  i_priority=High  i=0 A  i_nominal_specify=off  i_nominal_unit=A  i_nominal_value=1  v_specify=off  v_priority=High  v=0 V  v_nominal_specify=off  v_nominal_unit=V  v_nominal_value=1  t_specify=off  t_priority=High  t=0 N*m  t_nominal_specify=off  t_nominal_unit=N*m  t_nominal_value=1  w_specify=off  w_priority=High  w=0 rad/s  w_nominal_specify=off  w_nominal_unit=rad/s  w_nominal_value=1
      settings: SourceProductBaseCode=PW,SS,VE
  Thermal Resistor : fl_lib/Electrical/Electrical Elements/Thermal Resistor  R0=1 Ohm  T0=298.15 K  alpha=50e-6 1/K  tc=30 s  K_d=100 W/K  T_specify=off  T_priority=High  T=300 K  T_nominal_specify=off  T_nominal_unit=K  T_nominal_value=1
      settings: SourceProductBaseCode=PW,SS,VE  InternalSimscapePortConfiguration="{\"Bottom\":[],\"Left\":[{\"id\":\"H\",\"label\":\"H\",\"type\":\"foundation.thermal.thermal\"},{\"id\":\"p\",\"label\":\"+\",\"type\":\"foundation.electrical.electrical\"}],\"Right\":[{\"id\":\"n\",\"label\":\"-\",\"type\":\"foundation.electrical.electrical\"}],\"Top\":[]}"
  V+ : PMIOPort  Side=Left
  R : PMIOPort  Port=2  Side=Right
  C : PMIOPort  Port=3  Side=Right
  V- : PMIOPort  Port=4  Side=Left
  H : PMIOPort  Port=5  Side=Left
  connections:
  Thermal Resistor/RConn1 -- Rotational Electromechanical Converter/LConn1
  V-/RConn1 -- Rotational Electromechanical Converter/RConn1
  Thermal Resistor/LConn2 -- V+/RConn1
  Rotational Electromechanical Converter/LConn2 -- Inertia/LConn1 -- R/RConn1
  Rotational Electromechanical Converter/RConn2 -- C/RConn1
  H/RConn1 -- Thermal Resistor/LConn1

== system ssc_auto_ev_20b/Step 4: Deployment Model/Vehicle and drive @100Hz/Motor Drive/Motor Torque Controller 1 (System-Level Representation) ==
  Controlled Current Source : fl_lib/Electrical/Electrical Sources/Controlled Current Source
      settings: SourceProductBaseCode=PW,SS,VE
  +1 : PMIOPort  Side=Right
  +2 : PMIOPort  Port=2  Side=Left
  -1 : PMIOPort  Port=3  Side=Right
  -2 : PMIOPort  Port=4  Side=Left
  iRef : PMIOPort  Port=5  Side=Left
  connections:
  iRef/RConn1 -- Controlled Current Source/RConn1
  -2/RConn1 -- -1/RConn1
  Controlled Current Source/LConn1 -- +2/RConn1
  Controlled Current Source/RConn2 -- +1/RConn1

== system ssc_auto_ev_20b/Step 4: Deployment Model/Vehicle and drive @100Hz/Motor Drive/Motor Torque Controller 1 (System-Level Representation)1 ==
  Controlled Current Source : fl_lib/Electrical/Electrical Sources/Controlled Current Source
      settings: SourceProductBaseCode=PW,SS,VE
  +1 : PMIOPort  Side=Right
  +2 : PMIOPort  Port=2  Side=Left
  -1 : PMIOPort  Port=3  Side=Right
  -2 : PMIOPort  Port=4  Side=Left
  iRef : PMIOPort  Port=5  Side=Left
  connections:
  Controlled Current Source/RConn2 -- +1/RConn1
  Controlled Current Source/LConn1 -- +2/RConn1
  -2/RConn1 -- -1/RConn1
  iRef/RConn1 -- Controlled Current Source/RConn1

== system ssc_auto_ev_20b/Step 4: Deployment Model/Vehicle and drive @100Hz/Motor Drive/Sensing wMotor ==
  PS-Simulink Converter : nesl_utility/PS-Simulink Converter  PhysicalDomain=network_engine_domain  SubClassName=ps_output  LeftPortType=input  RightPortType=output  PseudoPeriodic=off  Frequencies=[]  Unit=rad/s  AffineConversion=off
      settings: SourceProductBaseCode=SS,PW,VE
  PS : PMIOPort  Side=Left
  SL : Outport  VectorParamsAs1DForOutWhenUnconnected=off
  wires:
  PS-Simulink Converter/1 -> SL/1
  connections:
  PS/RConn1 -- PS-Simulink Converter/LConn1

== system ssc_auto_ev_20b/Step 4: Deployment Model/Vehicle and drive @100Hz/Port 1 Interface1/Interface ==
  through1 : Inport
  through2 : Inport  Port=2
  Continuous : Subsystem  VariantControl=Continuous
  Discrete : Subsystem  VariantControl=Discrete
  across2 : Outport
  across1 : Outport  Port=2

== system ssc_auto_ev_20b/Step 4: Deployment Model/Vehicle and drive @100Hz/Port 1 Interface2/Interface ==
  through1 : Inport
  through2 : Inport  Port=2
  Continuous : Subsystem  VariantControl=Continuous
  Discrete : Subsystem  VariantControl=Discrete
  across2 : Outport
  across1 : Outport  Port=2

== system ssc_auto_ev_20b/Step 4: Deployment Model/Vehicle and drive @100Hz/Port 1 Interface3/Interface ==
  through1 : Inport
  across2 : Inport  Port=2
  Continuous : Subsystem  VariantControl=Continuous
  Discrete : Subsystem  VariantControl=Discrete
  through2 : Outport
  across1 : Outport  Port=2

== system ssc_auto_ev_20b/Step 4: Deployment Model/Vehicle and drive @100Hz/Vehicle Dynamics/Brake Torque ==
  Pedal : Inport
  Force for max pedal deflection : Gain  Gain=force_max_pedal
  Ideal Torque Source : fl_lib/Mechanical/Mechanical Sources/Ideal Torque Source
      settings: SourceProductBaseCode=PW,SS,VE
  MRRef : fl_lib/Mechanical/Rotational Elements/Mechanical Rotational Reference
      settings: SourceProductBaseCode=PW,SS,VE
  Motion Sensor : fl_lib/Mechanical/Mechanical Sensors/Ideal Rotational Motion Sensor  wrap_angle=simscape.enum.onoff.off  offset=0 rad
      settings: SourceProductBaseCode=PW,SS,VE
  PS Product : fl_lib/Physical Signals/Functions/PS Product
      settings: SourceProductBaseCode=PW,SS,VE
  Simulink-PS Converter1 : nesl_utility/Simulink-PS Converter  PhysicalDomain=network_engine_domain  SubClassName=ps_input  LeftPortType=input  RightPortType=output  PseudoPeriodic=off  Frequencies=[]  NoiseDistribution=none  NoiseParameters=[]  Unit=N*m  AffineConversion=off  FilteringAndDerivatives=zero  SimscapeFilterOrder=1  InputFilterTimeConstant=0.001  UdotUserProvided=1
      settings: SourceProductBaseCode=SS,PW,VE
  Smooth Sign : Subsystem
  Torque per unit brake pedal force : Gain  Gain=braking_torque_to_pedal_force_ratio
  R : PMIOPort  Side=Right
  wires:
  Torque per unit brake pedal force/1 -> Simulink-PS Converter1/1
  Pedal/1 -> Force for max pedal deflection/1
  Force for max pedal deflection/1 -> Torque per unit brake pedal force/1
  connections:
  Smooth Sign/RConn1 -- PS Product/LConn1
  Motion Sensor/RConn1 -- MRRef/LConn1 -- Ideal Torque Source/RConn2
  Ideal Torque Source/LConn1 -- Motion Sensor/LConn1 -- R/RConn1
  PS Product/RConn1 -- Ideal Torque Source/RConn1
  PS Product/LConn2 -- Simulink-PS Converter1/RConn1
  Smooth Sign/LConn1 -- Motion Sensor/RConn2

== system ssc_auto_ev_20b/Step 4: Deployment Model/Vehicle and drive @100Hz/Vehicle Dynamics/Drag and Gravity ==
  beta : Inport
  vW : Inport  Port=2
  " M*g " : fl_lib/Physical Signals/Functions/PS Gain  gain=vehicle_mass*gravity kg*m/s^2
      settings: SourceProductBaseCode=PW,SS,VE
  " tanh(u) " : fl_lib/Physical Signals/Functions/PS Math Function  fcn_choice=foundation.enum.math_function.tanh
      settings: SourceProductBaseCode=PW,SS,VE
  -1 : fl_lib/Physical Signals/Functions/PS Gain  gain=-1
      settings: SourceProductBaseCode=PW,SS,VE
  0.5*Cd*density*area : fl_lib/Physical Signals/Functions/PS Gain  gain=0.5*drag_coefficient*air_density*area kg/m^3*m^2
      settings: SourceProductBaseCode=PW,SS,VE
  1s/m : fl_lib/Physical Signals/Functions/PS Gain  gain=1 1/(m/s)
      settings: SourceProductBaseCode=PW,SS,VE
  M*g : fl_lib/Physical Signals/Functions/PS Gain  gain=vehicle_mass*gravity kg*m/s^2
      settings: SourceProductBaseCode=PW,SS,VE
  PS Add : fl_lib/Physical Signals/Functions/PS Add
      settings: SourceProductBaseCode=PW,SS,VE
  PS Gain : fl_lib/Physical Signals/Functions/PS Gain  gain=1 1/(m/s)
      settings: SourceProductBaseCode=PW,SS,VE
  PS Product : fl_lib/Physical Signals/Functions/PS Product
      settings: SourceProductBaseCode=PW,SS,VE
  PS Product2 : fl_lib/Physical Signals/Functions/PS Product
      settings: SourceProductBaseCode=PW,SS,VE
  PS Subtract : fl_lib/Physical Signals/Functions/PS Subtract
      settings: SourceProductBaseCode=PW,SS,VE
  Rolling resistance (fraction of normal force) : fl_lib/Physical Signals/Functions/PS Gain  gain=rolling_res_ratio
      settings: SourceProductBaseCode=PW,SS,VE
  Simulink-PS Converter2 : nesl_utility/Simulink-PS Converter  PhysicalDomain=network_engine_domain  SubClassName=ps_input  LeftPortType=input  RightPortType=output  PseudoPeriodic=off  Frequencies=[]  NoiseDistribution=none  NoiseParameters=[]  Unit=m/s  AffineConversion=off  FilteringAndDerivatives=zero  SimscapeFilterOrder=1  InputFilterTimeConstant=0.001  UdotUserProvided=1
      settings: SourceProductBaseCode=SS,PW,VE
  Simulink-PS Converter3 : nesl_utility/Simulink-PS Converter  PhysicalDomain=network_engine_domain  SubClassName=ps_input  LeftPortType=input  RightPortType=output  PseudoPeriodic=off  Frequencies=[]  NoiseDistribution=none  NoiseParameters=[]  Unit=deg  AffineConversion=off  FilteringAndDerivatives=zero  SimscapeFilterOrder=1  InputFilterTimeConstant=0.001  UdotUserProvided=1
      settings: SourceProductBaseCode=SS,PW,VE
  cos(u) : fl_lib/Physical Signals/Functions/PS Math Function  fcn_choice=foundation.enum.math_function.cos
      settings: SourceProductBaseCode=PW,SS,VE
  sin(u) : fl_lib/Physical Signals/Functions/PS Math Function  fcn_choice=foundation.enum.math_function.sin
      settings: SourceProductBaseCode=PW,SS,VE
  tanh(u) : fl_lib/Physical Signals/Functions/PS Math Function  fcn_choice=foundation.enum.math_function.tanh
      settings: SourceProductBaseCode=PW,SS,VE
  u^2 : fl_lib/Physical Signals/Functions/PS Math Function  fcn_choice=foundation.enum.math_function.square
      settings: SourceProductBaseCode=PW,SS,VE
  vV : PMIOPort  Side=Left
  F : PMIOPort  Port=2  Side=Left
  F2 : PMIOPort  Port=3  Side=Left
  wires:
  beta/1 -> Simulink-PS Converter3/1
  vW/1 -> Simulink-PS Converter2/1
  connections:
  " M*g "/LConn1 -- cos(u)/RConn1
  M*g/LConn1 -- sin(u)/RConn1
  Rolling resistance (fraction of normal force)/LConn1 -- " M*g "/RConn1
  M*g/RConn1 -- PS Add/LConn1
  sin(u)/LConn1 -- Simulink-PS Converter3/RConn1 -- cos(u)/LConn1
  PS Product2/LConn2 -- 0.5*Cd*density*area/RConn1
  " tanh(u) "/LConn1 -- PS Gain/RConn1
  0.5*Cd*density*area/LConn1 -- u^2/RConn1
  " tanh(u) "/RConn1 -- PS Product2/LConn1
  u^2/LConn1 -- PS Subtract/RConn1 -- PS Gain/LConn1
  tanh(u)/LConn1 -- 1s/m/RConn1
  PS Product/LConn1 -- tanh(u)/RConn1
  -1/RConn1 -- F2/RConn1
  PS Add/RConn1 -- -1/LConn1
  PS Product/RConn1 -- PS Add/LConn2
  PS Product/LConn2 -- Rolling resistance (fraction of normal force)/RConn1
  PS Product2/RConn1 -- F/RConn1
  Simulink-PS Converter2/RConn1 -- PS Subtract/LConn2
  PS Subtract/LConn1 -- 1s/m/LConn1 -- vV/RConn1

== system ssc_auto_ev_20b/Step 4: Deployment Model/Vehicle and drive @100Hz/Vehicle Dynamics/Sensing Speed ==
  MTRef : fl_lib/Mechanical/Translational Elements/Mechanical Translational Reference
      settings: SourceProductBaseCode=PW,SS,VE
  Motion Sensor : fl_lib/Mechanical/Mechanical Sensors/Ideal Translational Motion Sensor  offset=0 m
      settings: SourceProductBaseCode=PW,SS,VE
  R : PMIOPort  Side=Left
  w : PMIOPort  Port=2  Side=Right
  connections:
  R/RConn1 -- Motion Sensor/LConn1
  MTRef/LConn1 -- Motion Sensor/RConn1
  Motion Sensor/RConn2 -- w/RConn1

== system ssc_auto_ev_20b/Step 2: Multirate Model/Battery Thermal Mass/Port 1 Interface/Interface/Continuous ==
  through2 : Inport
  through1 : Inport  Port=2
  1/thermalMass : Gain  Gain=1/thermalMass  SaturateOnIntegerOverflow=on  OutDataTypeStr=Inherit: Same as input  ParamDataTypeStr=Inherit: Same as input
  Integrator : Integrator  InitialCondition=T0
  Prediction : Subsystem  Commented=through  mask(Prediction (discrete->continuous)){h2=h2}
      mask prompts: h2 "physmod:simscape:couplers:SimscapeNetworkCouplersLib:PortUDiscreteSampleTimes_MP"
      mask help: physmod:simscape:couplers:SimscapeNetworkCouplersLib:Predictiondiscretecontinuous_MD
  Smoothing : Subsystem  Commented=through  mask(Smoothing (continuous->discrete)){tsSmoothing=tsSmoothing, smoothing0=T0}
      mask prompts: tsSmoothing "physmod:simscape:couplers:SimscapeNetworkCouplersLib:SmoothingTimeConstants_MP"; smoothing0 "physmod:simscape:couplers:SimscapeNetworkCouplersLib:InitialOutput_MP"
      mask help: physmod:simscape:couplers:SimscapeNetworkCouplersLib:Smoothingcontinuousdiscrete_MD
  Sum : Sum  InputSameDT=on  SaturateOnIntegerOverflow=on  OutDataTypeStr=Inherit: Same as first input
  across2 : Outport
  across1 : Outport  Port=2
  wires:
  through2/1 -> Prediction/1(u)
  through1/1 -> Sum/1
  Prediction/1(y) -> Sum/2
  Smoothing/1(y) -> across2/1
  Sum/1 -> 1/thermalMass/1
  1/thermalMass/1 -> Integrator/1
  Integrator/1 -> across1/1, Smoothing/1(u)

== system ssc_auto_ev_20b/Step 2: Multirate Model/Battery Thermal Mass/Port 1 Interface/Interface/Discrete ==
  through2 : Inport
  through1 : Inport  Port=2
  1/thermalMass : Gain  Gain=1/thermalMass  SaturateOnIntegerOverflow=on  OutDataTypeStr=Inherit: Same as input  ParamDataTypeStr=Inherit: Same as input
  Integrator : DiscreteIntegrator  InitialCondition=T0  SampleTime=h1  ICPrevOutput=DiscIntNeverNeededParam  ICPrevScaledInput=DiscIntNeverNeededParam
  Prediction : Subsystem  Commented=through  mask(Prediction (slow->fast)){h2=h2, h1=h1}
      mask prompts: h2 "physmod:simscape:couplers:SimscapeNetworkCouplersLib:PortUDiscreteSampleTimes_MP"; h1 "physmod:simscape:couplers:SimscapeNetworkCouplersLib:PortYDiscreteSampleTimes_MP"
      mask help: physmod:simscape:couplers:SimscapeNetworkCouplersLib:Predictionslowfast_MD
  Smoothing : Subsystem  Commented=through  mask(Smoothing (fast->slow)){nSmooth=nSmooth, h1=h1, smoothing0=T0}
      mask prompts: nSmooth "physmod:simscape:couplers:SimscapeNetworkCouplersLib:NumberOfSamplesOverWhichToSmooth_MP"; h1 "physmod:simscape:couplers:SimscapeNetworkCouplersLib:PortUDiscreteSampleTimes_MP"; smoothing0 "physmod:simscape:couplers:SimscapeNetworkCouplersLib:InitialOutput_MP"
      mask help: physmod:simscape:couplers:SimscapeNetworkCouplersLib:Smoothingfastslow_MD
  Sum : Sum  InputSameDT=on  SaturateOnIntegerOverflow=on  OutDataTypeStr=Inherit: Same as first input
  across2 : Outport
  across1 : Outport  Port=2
  wires:
  through1/1 -> Sum/1
  through2/1 -> Prediction/1(u)
  Prediction/1(y) -> Sum/2
  Smoothing/1(y) -> across2/1
  Integrator/1 -> across1/1, Smoothing/1(u)
  Sum/1 -> 1/thermalMass/1
  1/thermalMass/1 -> Integrator/1
